simulink model "Lab_3_ADCDAC_System"  (R2024a)
settings: Solver=VariableStepAuto  StartTime=0.0  StopTime=10.0  RelTol=1e-3
libraries: dspquant2 x2, dspfdesign x1, dspsigops x1
settings Model: Creator=pyrpo  LastModifiedBy=pyrpo

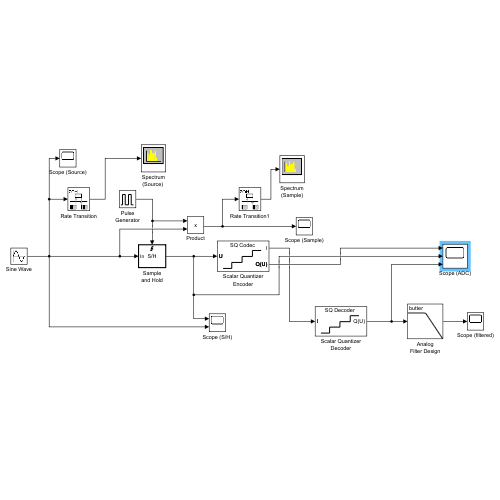
[thumbnail: Simulink's stored preview of the top-level diagram]
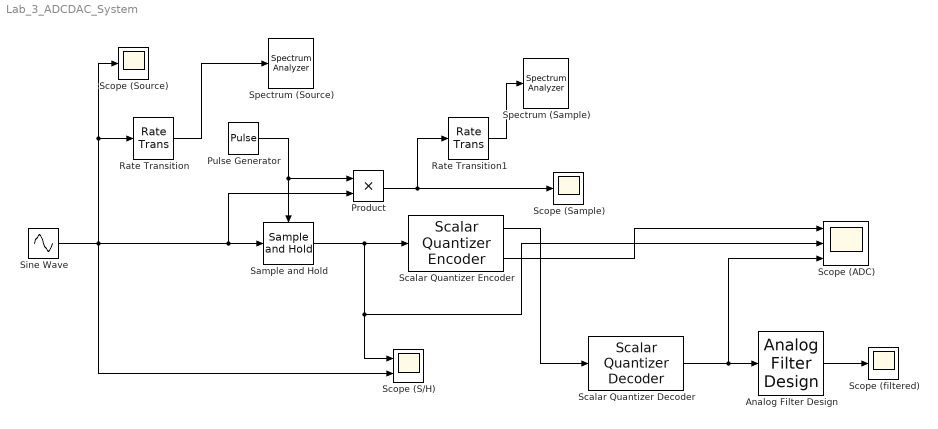
== system Lab_3_ADCDAC_System ==
  Analog Filter Design : dspfdesign/Analog Filter Design  method=Butterworth  filttype=Lowpass  N=20  Wlo=500*2*pi  Whi=80  Rp=2  Rs=40
  Product : Product
  Pulse Generator : DiscretePulseGenerator  PulseType=Time based  Period=0.001/8  PulseWidth=50
  Rate Transition : RateTransition  OutPortSampleTime=1e-5
  Rate Transition1 : RateTransition  OutPortSampleTime=1e-5
  Sample and Hold : dspsigops/Sample and Hold  trig=Rising edge  initCond=0  latchinput=off
  Scalar Quantizer Decoder : dspquant2/Scalar Quantizer Decoder  invalidin=Error  CBsource=Specify via dialog  codebook=[-1.5:1:1.5]  dataType=double  isSigned=on  wordLen=16  udDataType=sfix(16)  fracBitsMode=Best precision  numFracBits=11  OutDataTypeStr=double  LastOutDataTypeStr=double
  Scalar Quantizer Encoder : dspquant2/Scalar Quantizer Encoder  paramSrc=Specify via dialog  partType=Bounded  BBoundary=[-2:2]  UBoundary=[2:9]  SearchMethod=Linear  tieBreakRule=Choose the higher index  outQU=on  outQError=off  codebook=[-1.5:1:1.5]  outStatus=off  invalidin=Clip  idtype=int32  roundingMode=Floor  overflowMode=off
  Scope (ADC) : Scope  NumInputPorts=3
  Scope (S/H) : Scope  NumInputPorts=2
  Scope (Sample) : Scope
  Scope (Source) : Scope
  Scope (filtered) : Scope
  Sine Wave : Sin  Amplitude=2  Frequency=500*2*pi  SampleTime=0
  Spectrum (Sample) : SpectrumAnalyzer  WindowPosition=[-36.000000,-78.000000,1099.000000,596.000000,]  ScopeFrameLocation=window  Span=99999.99999999999  StartFrequency=-49999.99999999999  StopFrequency=49999.99999999999  YLimits=[-229.38580018,52.50960302]
  "Spectrum (Source) " : SpectrumAnalyzer  WindowPosition=[-7.000000,-27.000000,1099.000000,596.000000,]  ScopeFrameLocation=window  YLimits=[-262.76280778,62.52919623]
  wires:
  Sine Wave/1 -> Scope (S/H)/2, Scope (Source)/1, Rate Transition/1, Product/2, Sample and Hold/1
  Rate Transition/1 -> "Spectrum (Source) "/1
  Pulse Generator/1 -> Sample and Hold/Trigger, Product/1
  Product/1 -> Rate Transition1/1, Scope (Sample)/1
  Rate Transition1/1 -> Spectrum (Sample)/1
  Sample and Hold/1 -> Scalar Quantizer Encoder/1, Scope (S/H)/1, Scope (ADC)/2
  Scalar Quantizer Encoder/1 -> Scalar Quantizer Decoder/1
  Scalar Quantizer Decoder/1 -> Scope (ADC)/3, Analog Filter Design/1
  Scalar Quantizer Encoder/2 -> Scope (ADC)/1
  Analog Filter Design/1 -> Scope (filtered)/1
